simulink model "on_off_control_oven_2014"  (R2014a)
settings: Solver=ode45  SolverMode=SingleTasking  StartTime=0.0  StopTime=1000  RelTol=1e-3
settings Model: CovMetricSettings=dwe  CovHtmlReporting=off  covSaveCumulativeToWorkspaceVar=off  CovSaveSingleToWorkspaceVar=off  CovExternalEMLEnable=on  CovSFcnEnable=on  Creator=root  LastModifiedBy=root
settings DataIOCC: LimitDataPoints=off  SaveFormat=StructureWithTime
settings DebuggingCC: MergeDetectMultiDrivingBlocksExec=error  SolverPrmCheckMsg=none  FrameProcessingCompatibilityMsg=error  SFUnexpectedBacktrackingDiag=error  SFNoUnconditionalDefaultTransitionDiag=error
settings HardwareCC: ProdBitPerPointer=64  ProdLargestAtomicFloat=Float  ProdIntDivRoundTo=Zero  ProdEndianess=LittleEndian  ProdHWDeviceType=Specified
settings ModelReferenceCC: PropagateSignalLabelsOutOfModel=on
settings SFSimCC: SimUseLocalCustomCode=on
settings RTWCC: RTWUseLocalCustomCode=on
settings GRTTargetCC: TargetLangStandard=C99 (ISO)  GeneratePreprocessorConditionals=Use local settings

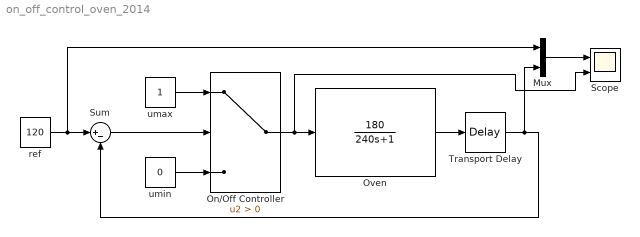
== system on_off_control_oven_2014 ==
  Mux : Mux  Inputs=2
  On/Off Controller : Switch  Criteria=u2 > Threshold
  Oven : TransferFcn  Numerator=[180]  Denominator=[240 1]
  Scope : Scope  NumInputPorts=2
      settings: TimeRange=auto  MaxDataPoints=5000  SaveToWorkspace=off  SaveName=ScopeData  YMin=-15.60108~-0.125  YMax=140.40972~1.125  SampleTime=-1
  Sum : Sum  Inputs=|+-
  Transport Delay : TransportDelay  DelayTime=30
  ref : Constant  Value=120
  "umax " : Constant
  umin : Constant  Value=0
  wires:
  Oven/1 -> Transport Delay/1
  Sum/1 -> On/Off Controller/2
  "umax "/1 -> On/Off Controller/1
  ref/1 -> Mux/1, Sum/1
  umin/1 -> On/Off Controller/3
  On/Off Controller/1 -> Scope/2, Oven/1
  Mux/1 -> Scope/1
  Transport Delay/1 -> Mux/2, Sum/2
